simulink model "omav_old_allocation"  (R2020a)
settings: Solver=VariableStepAuto  StartTime=0.0  StopTime=15  RelTol=1e-3
undefined symbols (not defined in the file): params
libraries: simulink x12, vrlib x2
settings Model: Creator=daniel  LastModifiedBy=daniel

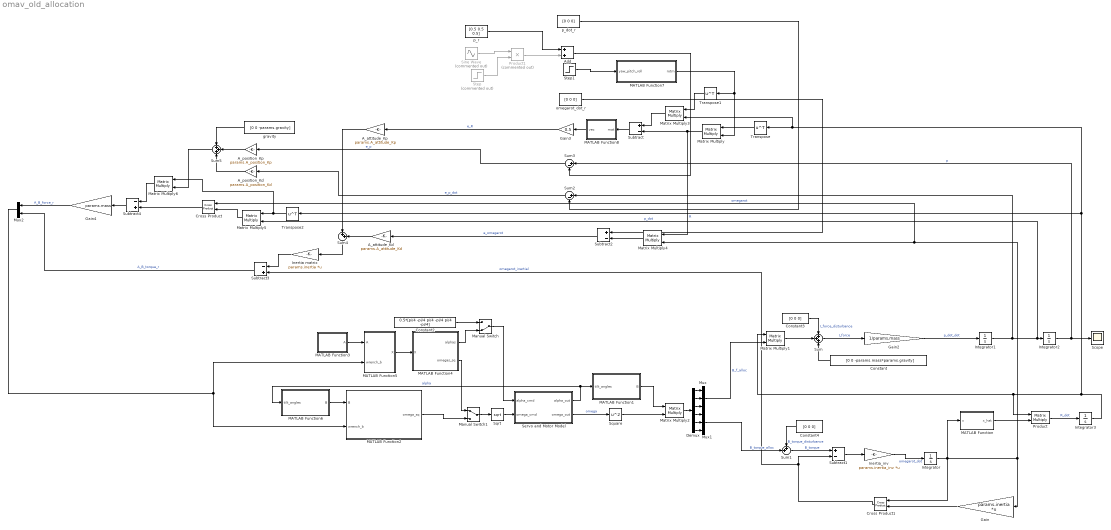
== system omav_old_allocation ==
  A_attitude_Kd : Gain  Gain=params.A_attitude_Kd
  A_attitude_Kp : Gain  Gain=params.A_attitude_Kp
  A_position_Kd : Gain  Gain=params.A_position_Kd
  A_position_Kp : Gain  Gain=params.A_position_Kp
  Add : Sum
  Constant : Constant  Value=[0 0 -params.mass*params.gravity]
  Constant2 : Constant  Value=0.5*[pi/4 -pi/4 pi/4 -pi/4 pi/4 -pi/4]
  Constant3 : Constant  Value=[0 0 0]
  Constant4 : Constant  Value=[0 0 0]
  Cross Product : vrlib/Utilities/Cross Product
  Cross Product1 : vrlib/Utilities/Cross Product
  Demux : Demux  Outputs=6
  Gain : Gain  Gain=params.inertia  Multiplication=Matrix(K*u) (u vector)
  Gain2 : Gain  Gain=1/params.mass
  Gain3 : Gain  Gain=0.5
  Gain4 : Gain  Gain=params.mass
  Inertia matrix : Gain  Gain=params.inertia  Multiplication=Matrix(K*u) (u vector)
  Inertia_inv : Gain  Gain=params.inertia_inv  Multiplication=Matrix(K*u) (u vector)
  Integrator : Integrator
  Integrator1 : Integrator
  Integrator2 : Integrator
  Integrator3 : Integrator  InitialCondition=[1 0 0;0 1 0;0 0 1]
  MATLAB Function : MATLAB Function  TreatAsAtomicUnit=on
  MATLAB Function1 : MATLAB Function  TreatAsAtomicUnit=on
  MATLAB Function2 : MATLAB Function  TreatAsAtomicUnit=on
  MATLAB Function3 : MATLAB Function  TreatAsAtomicUnit=on
  MATLAB Function4 : MATLAB Function  TreatAsAtomicUnit=on
  MATLAB Function5 : MATLAB Function  TreatAsAtomicUnit=on
  MATLAB Function6 : MATLAB Function  TreatAsAtomicUnit=on
  MATLAB Function7 : MATLAB Function  TreatAsAtomicUnit=on
  MATLAB Function8 : MATLAB Function  TreatAsAtomicUnit=on
  Manual Switch : ManualSwitch  CurrentSetting=0
  Manual Switch1 : ManualSwitch
  Matrix Multiply{,1..6} (7 alike) : Product  Multiplication=Matrix(*)
  Mux : Mux  Inputs=3
  Mux1 : Mux  Inputs=3
  Mux2 : Mux  Inputs=2
  Product : Product  Multiplication=Matrix(*)  OutMin=0
  Product1 : Product  Commented=on
  Scope : Scope
  Servo and Motor Model : Subsystem
  Sine Wave : Sin  Commented=on  Amplitude=[0.01 0 0]  Frequency=5  SampleTime=0
  Sqrt : Sqrt  SaturateOnIntegerOverflow=on
  Square : Math  Operator=square  SaturateOnIntegerOverflow=on
  Step : Step  Commented=on  Time=3  SampleTime=0
  Step1 : Step  Time=5  Before=[0 0 0]  After=[0 pi/2 0]  SampleTime=0
  Subtract : Sum  Inputs=+-
  Subtract1 : Sum  Inputs=+-
  Subtract2 : Sum  Inputs=+-
  Subtract3 : Sum  Inputs=-+
  Subtract4 : Sum  Inputs=-+
  Sum : Sum  Inputs=+++
  Sum1 : Sum  Inputs=++|
  Sum2 : Sum  Inputs=|+-
  Sum3 : Sum  Inputs=|+-
  Sum4 : Sum  Inputs=|++
  Sum5 : Sum  Inputs=+++
  Transpose : Math  Operator=transpose  SaturateOnIntegerOverflow=on
  Transpose1 : Math  Operator=transpose  SaturateOnIntegerOverflow=on
  Transpose2 : Math  Operator=transpose  SaturateOnIntegerOverflow=on
  gravity : Constant  Value=[0 0 -params.gravity]
  omegarot_dot_r : Constant  Value=[0 0 0]
  p_dot_r : Constant  Value=[0 0 0]
  p_r : Constant  Value=[0.5 0.5 0.5]
  wires:
  Integrator1/1 -> Matrix Multiply5/2, Integrator2/1, Sum2/1  "p_dot"
  Integrator2/1 -> Sum3/1, Scope/1  "p"
  Gain2/1 -> Integrator1/1  "p_dot_dot"
  Integrator/1 -> Cross Product/1, Matrix Multiply4/2, Gain/1, MATLAB Function/1(x), Cross Product1/1  "omegarot"
  Subtract1/1 -> Inertia_inv/1
  Gain/1 -> Cross Product1/2
  Cross Product1/1 -> Subtract3/2, Subtract1/2  "omegarot_inertial"
  Inertia_inv/1 -> Integrator/1  "omegarot_dot"
  Mux1/1 -> Sum1/2  "B_torque_alloc"
  Sum/1 -> Gain2/1  "I_force"
  MATLAB Function/1(x_hat) -> Product/2
  Integrator3/1 -> Matrix Multiply3/2, Transpose/1, Transpose2/1, Product/1, Matrix Multiply1/1  "R"
  Product/1 -> Integrator3/1  "R_dot"
  Constant3/1 -> Sum/1  "I_force_disturbance"
  Mux/1 -> Matrix Multiply1/2  "B_f_alloc"
  Matrix Multiply1/1 -> Sum/2
  Constant/1 -> Sum/3
  Sum1/1 -> Subtract1/1  "B_torque"
  Constant4/1 -> Sum1/1  "B_torque_disturbance"
  MATLAB Function1/1(B) -> Matrix Multiply2/1
  Matrix Multiply2/1 -> Demux/1
  Demux/1 -> Mux/1
  Demux/2 -> Mux/2
  Demux/3 -> Mux/3
  Demux/5 -> Mux1/2
  Demux/4 -> Mux1/1
  Demux/6 -> Mux1/3
  Servo and Motor Model/1(alpha_out) -> MATLAB Function6/1(tilt_angles), MATLAB Function1/1(tilt_angles)  "alpha"
  Servo and Motor Model/2(omega_out) -> Square/1  "omega"
  Square/1 -> Matrix Multiply2/2
  MATLAB Function2/1(omega_sq) -> Manual Switch1/2
  Sqrt/1 -> Servo and Motor Model/2(omega_cmd)
  MATLAB Function3/1(A) -> MATLAB Function5/1(A)
  MATLAB Function5/1(X) -> MATLAB Function4/1(X)
  MATLAB Function6/1(B) -> MATLAB Function2/1(B)
  MATLAB Function4/1(alphas) -> Manual Switch/2
  Manual Switch/1 -> Servo and Motor Model/1(alpha_cmd)
  Constant2/1 -> Manual Switch/1
  p_dot_r/1 -> Sum2/2
  Sum2/1 -> A_position_Kd/1  "e_p_dot"
  Sum3/1 -> A_position_Kp/1  "e_p"
  Add/1 -> Sum3/2
  Step1/1 -> MATLAB Function7/1(yaw_pitch_roll)
  MATLAB Function7/1(rotm) -> Matrix Multiply/2, Transpose1/1
  Matrix Multiply/1 -> Subtract/2, Matrix Multiply4/1
  Transpose/1 -> Matrix Multiply/1
  Transpose1/1 -> Matrix Multiply3/1
  Matrix Multiply3/1 -> Subtract/1
  Subtract/1 -> MATLAB Function8/1(mat)
  MATLAB Function8/1(vec) -> Gain3/1
  Gain3/1 -> A_attitude_Kp/1  "e_R"
  omegarot_dot_r/1 -> Subtract2/1
  Matrix Multiply4/1 -> Subtract2/2
  Subtract2/1 -> A_attitude_Kd/1  "e_omegarot"
  A_attitude_Kd/1 -> Sum4/2
  A_attitude_Kp/1 -> Sum4/1
  Sum4/1 -> Inertia matrix/1
  Inertia matrix/1 -> Subtract3/1
  Subtract3/1 -> Mux2/2  "A_B_torque_r"
  Transpose2/1 -> Matrix Multiply6/1, Matrix Multiply5/1
  Matrix Multiply5/1 -> Cross Product/2
  A_position_Kp/1 -> Sum5/2
  gravity/1 -> Sum5/1
  A_position_Kd/1 -> Sum5/3
  Sum5/1 -> Matrix Multiply6/2
  Matrix Multiply6/1 -> Subtract4/1
  Cross Product/1 -> Subtract4/2
  Subtract4/1 -> Gain4/1
  Gain4/1 -> Mux2/1  "A_B_force_r"
  Mux2/1 -> MATLAB Function5/2(wrench_b), MATLAB Function2/2(wrench_b)
  Manual Switch1/1 -> Sqrt/1
  MATLAB Function4/2(omegas_sq) -> Manual Switch1/1
  Step/1 -> Product1/2
  Sine Wave/1 -> Product1/1
  Product1/1 -> Add/2
  p_r/1 -> Add/1

== system omav_old_allocation/Servo and Motor Model ==
  alpha_cmd : Inport
  omega_cmd : Inport  Port=2
  all_rotors_subsystem1 : Subsystem
      mask Display: image('images/brushless.JPG'); % Use "Edit Image" on toolstrip to change.
  all_servos_subsystem1 : Subsystem
      mask Display: image('images/servo.jpg'); % Use "Edit Image" on toolstrip to change.
  alpha_out : Outport
  omega_out : Outport  Port=2
  wires:
  alpha_cmd/1 -> all_servos_subsystem1/1(alphas_cmd)  "alpha_cmd"
  all_rotors_subsystem1/1(omegas_out) -> omega_out/1  "omega_out"
  all_servos_subsystem1/1(alphas_out) -> alpha_out/1  "alpha_out"
  omega_cmd/1 -> all_rotors_subsystem1/1(omegas_cmd)  "omega_cmd"

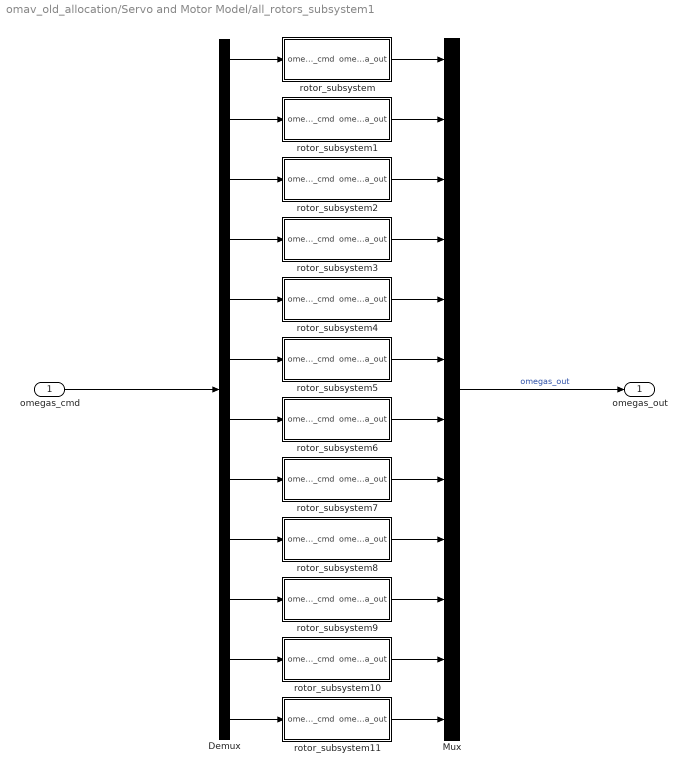
== system omav_old_allocation/Servo and Motor Model/all_rotors_subsystem1 ==
  omegas_cmd : Inport
  Demux : Demux  Outputs=12
  Mux : Mux  Inputs=12
  rotor_subsystem : Subsystem
  rotor_subsystem1 : Subsystem
  rotor_subsystem10 : Subsystem
  rotor_subsystem11 : Subsystem
  rotor_subsystem2 : Subsystem
  rotor_subsystem3 : Subsystem
  rotor_subsystem4 : Subsystem
  rotor_subsystem5 : Subsystem
  rotor_subsystem6 : Subsystem
  rotor_subsystem7 : Subsystem
  rotor_subsystem8 : Subsystem
  rotor_subsystem9 : Subsystem
  omegas_out : Outport
  wires:
  Demux/3 -> rotor_subsystem2/1(omega_cmd)
  rotor_subsystem10/1(omega_out) -> Mux/11
  rotor_subsystem7/1(omega_out) -> Mux/8
  rotor_subsystem2/1(omega_out) -> Mux/3
  rotor_subsystem1/1(omega_out) -> Mux/2
  Demux/2 -> rotor_subsystem1/1(omega_cmd)
  rotor_subsystem5/1(omega_out) -> Mux/6
  rotor_subsystem4/1(omega_out) -> Mux/5
  Demux/4 -> rotor_subsystem3/1(omega_cmd)
  rotor_subsystem6/1(omega_out) -> Mux/7
  Demux/8 -> rotor_subsystem7/1(omega_cmd)
  rotor_subsystem/1(omega_out) -> Mux/1
  rotor_subsystem3/1(omega_out) -> Mux/4
  rotor_subsystem11/1(omega_out) -> Mux/12
  rotor_subsystem8/1(omega_out) -> Mux/9
  Demux/11 -> rotor_subsystem10/1(omega_cmd)
  rotor_subsystem9/1(omega_out) -> Mux/10
  Demux/1 -> rotor_subsystem/1(omega_cmd)
  omegas_cmd/1 -> Demux/1
  Mux/1 -> omegas_out/1  "omegas_out"
  Demux/12 -> rotor_subsystem11/1(omega_cmd)
  Demux/10 -> rotor_subsystem9/1(omega_cmd)
  Demux/9 -> rotor_subsystem8/1(omega_cmd)
  Demux/7 -> rotor_subsystem6/1(omega_cmd)
  Demux/6 -> rotor_subsystem5/1(omega_cmd)
  Demux/5 -> rotor_subsystem4/1(omega_cmd)

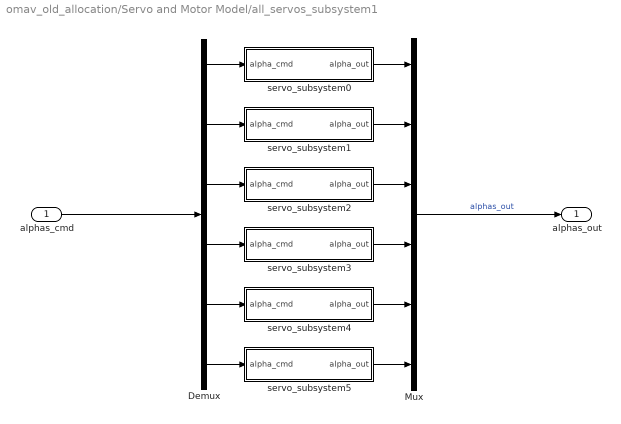
== system omav_old_allocation/Servo and Motor Model/all_servos_subsystem1 ==
  alphas_cmd : Inport
  Demux : Demux  Outputs=6
  Mux : Mux  Inputs=6
  servo_subsystem0 : Subsystem
  servo_subsystem1 : Subsystem
  servo_subsystem2 : Subsystem
  servo_subsystem3 : Subsystem
  servo_subsystem4 : Subsystem
  servo_subsystem5 : Subsystem
  alphas_out : Outport
  wires:
  alphas_cmd/1 -> Demux/1
  Demux/2 -> servo_subsystem1/1(alpha_cmd)
  servo_subsystem3/1(alpha_out) -> Mux/4
  servo_subsystem1/1(alpha_out) -> Mux/2
  Demux/4 -> servo_subsystem3/1(alpha_cmd)
  servo_subsystem4/1(alpha_out) -> Mux/5
  Demux/5 -> servo_subsystem4/1(alpha_cmd)
  Demux/1 -> servo_subsystem0/1(alpha_cmd)
  servo_subsystem2/1(alpha_out) -> Mux/3
  servo_subsystem5/1(alpha_out) -> Mux/6
  Demux/6 -> servo_subsystem5/1(alpha_cmd)
  Demux/3 -> servo_subsystem2/1(alpha_cmd)
  Mux/1 -> alphas_out/1  "alphas_out"
  servo_subsystem0/1(alpha_out) -> Mux/1

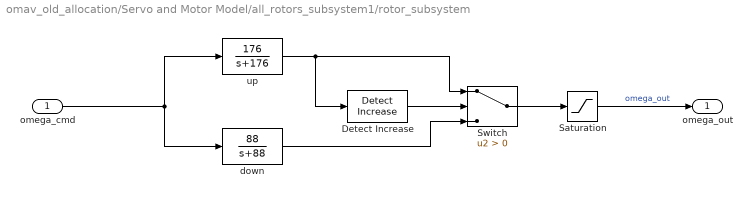
== system omav_old_allocation/Servo and Motor Model/all_rotors_subsystem1/rotor_subsystem ==
  omega_cmd : Inport
  Detect Increase : simulink/Logic and Bit Operations/Detect Increase  vinit=0.0  OutDataTypeStr=boolean
  Saturation : Saturate  UpperLimit=params.rotor_max  LowerLimit=0
  Switch : Switch  Criteria=u2 > Threshold
  down : TransferFcn  Numerator=[88]  Denominator=[1 88]
  up : TransferFcn  Numerator=[176]  Denominator=[1 176]
  omega_out : Outport
  wires:
  down/1 -> Switch/3
  up/1 -> Detect Increase/1, Switch/1
  omega_cmd/1 -> up/1, down/1
  Switch/1 -> Saturation/1
  Detect Increase/1 -> Switch/2
  Saturation/1 -> omega_out/1  "omega_out"

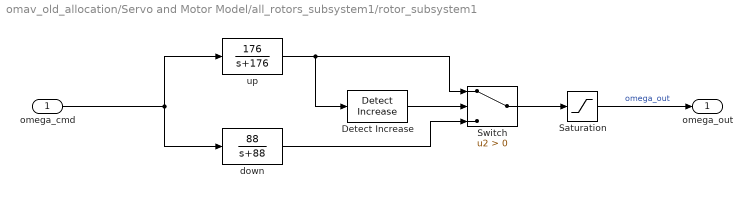
== system omav_old_allocation/Servo and Motor Model/all_rotors_subsystem1/rotor_subsystem1 ==
  omega_cmd : Inport
  Detect Increase : simulink/Logic and Bit Operations/Detect Increase  vinit=0.0  OutDataTypeStr=boolean
  Saturation : Saturate  UpperLimit=params.rotor_max  LowerLimit=0
  Switch : Switch  Criteria=u2 > Threshold
  down : TransferFcn  Numerator=[88]  Denominator=[1 88]
  up : TransferFcn  Numerator=[176]  Denominator=[1 176]
  omega_out : Outport
  wires:
  Saturation/1 -> omega_out/1  "omega_out"
  Detect Increase/1 -> Switch/2
  Switch/1 -> Saturation/1
  omega_cmd/1 -> down/1, up/1
  up/1 -> Switch/1, Detect Increase/1
  down/1 -> Switch/3

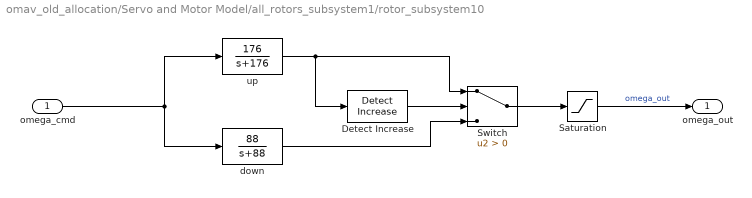
== system omav_old_allocation/Servo and Motor Model/all_rotors_subsystem1/rotor_subsystem10 ==
  omega_cmd : Inport
  Detect Increase : simulink/Logic and Bit Operations/Detect Increase  vinit=0.0  OutDataTypeStr=boolean
  Saturation : Saturate  UpperLimit=params.rotor_max  LowerLimit=0
  Switch : Switch  Criteria=u2 > Threshold
  down : TransferFcn  Numerator=[88]  Denominator=[1 88]
  up : TransferFcn  Numerator=[176]  Denominator=[1 176]
  omega_out : Outport
  wires:
  down/1 -> Switch/3
  up/1 -> Detect Increase/1, Switch/1
  omega_cmd/1 -> up/1, down/1
  Switch/1 -> Saturation/1
  Detect Increase/1 -> Switch/2
  Saturation/1 -> omega_out/1  "omega_out"

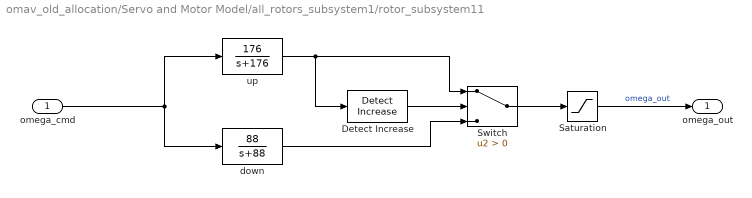
== system omav_old_allocation/Servo and Motor Model/all_rotors_subsystem1/rotor_subsystem11 ==
  omega_cmd : Inport
  Detect Increase : simulink/Logic and Bit Operations/Detect Increase  vinit=0.0  OutDataTypeStr=boolean
  Saturation : Saturate  UpperLimit=params.rotor_max  LowerLimit=0
  Switch : Switch  Criteria=u2 > Threshold
  down : TransferFcn  Numerator=[88]  Denominator=[1 88]
  up : TransferFcn  Numerator=[176]  Denominator=[1 176]
  omega_out : Outport
  wires:
  Saturation/1 -> omega_out/1  "omega_out"
  Detect Increase/1 -> Switch/2
  Switch/1 -> Saturation/1
  omega_cmd/1 -> down/1, up/1
  up/1 -> Switch/1, Detect Increase/1
  down/1 -> Switch/3

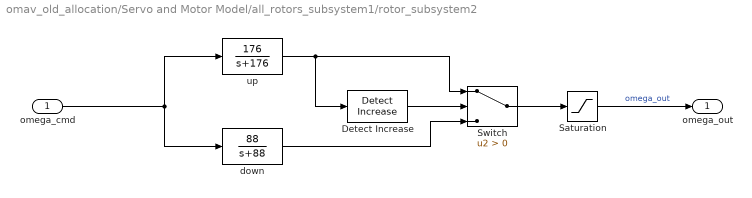
== system omav_old_allocation/Servo and Motor Model/all_rotors_subsystem1/rotor_subsystem2 ==
  omega_cmd : Inport
  Detect Increase : simulink/Logic and Bit Operations/Detect Increase  vinit=0.0  OutDataTypeStr=boolean
  Saturation : Saturate  UpperLimit=params.rotor_max  LowerLimit=0
  Switch : Switch  Criteria=u2 > Threshold
  down : TransferFcn  Numerator=[88]  Denominator=[1 88]
  up : TransferFcn  Numerator=[176]  Denominator=[1 176]
  omega_out : Outport
  wires:
  down/1 -> Switch/3
  up/1 -> Detect Increase/1, Switch/1
  omega_cmd/1 -> up/1, down/1
  Switch/1 -> Saturation/1
  Detect Increase/1 -> Switch/2
  Saturation/1 -> omega_out/1  "omega_out"

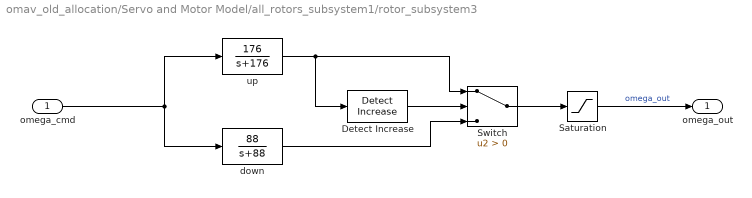
== system omav_old_allocation/Servo and Motor Model/all_rotors_subsystem1/rotor_subsystem3 ==
  omega_cmd : Inport
  Detect Increase : simulink/Logic and Bit Operations/Detect Increase  vinit=0.0  OutDataTypeStr=boolean
  Saturation : Saturate  UpperLimit=params.rotor_max  LowerLimit=0
  Switch : Switch  Criteria=u2 > Threshold
  down : TransferFcn  Numerator=[88]  Denominator=[1 88]
  up : TransferFcn  Numerator=[176]  Denominator=[1 176]
  omega_out : Outport
  wires:
  Saturation/1 -> omega_out/1  "omega_out"
  Detect Increase/1 -> Switch/2
  Switch/1 -> Saturation/1
  omega_cmd/1 -> down/1, up/1
  up/1 -> Switch/1, Detect Increase/1
  down/1 -> Switch/3

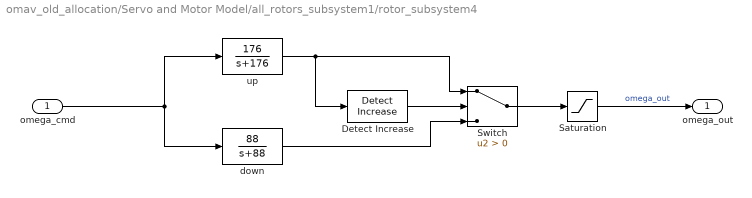
== system omav_old_allocation/Servo and Motor Model/all_rotors_subsystem1/rotor_subsystem4 ==
  omega_cmd : Inport
  Detect Increase : simulink/Logic and Bit Operations/Detect Increase  vinit=0.0  OutDataTypeStr=boolean
  Saturation : Saturate  UpperLimit=params.rotor_max  LowerLimit=0
  Switch : Switch  Criteria=u2 > Threshold
  down : TransferFcn  Numerator=[88]  Denominator=[1 88]
  up : TransferFcn  Numerator=[176]  Denominator=[1 176]
  omega_out : Outport
  wires:
  down/1 -> Switch/3
  up/1 -> Detect Increase/1, Switch/1
  omega_cmd/1 -> up/1, down/1
  Switch/1 -> Saturation/1
  Detect Increase/1 -> Switch/2
  Saturation/1 -> omega_out/1  "omega_out"

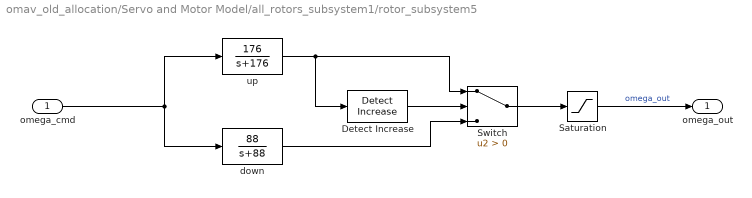
== system omav_old_allocation/Servo and Motor Model/all_rotors_subsystem1/rotor_subsystem5 ==
  omega_cmd : Inport
  Detect Increase : simulink/Logic and Bit Operations/Detect Increase  vinit=0.0  OutDataTypeStr=boolean
  Saturation : Saturate  UpperLimit=params.rotor_max  LowerLimit=0
  Switch : Switch  Criteria=u2 > Threshold
  down : TransferFcn  Numerator=[88]  Denominator=[1 88]
  up : TransferFcn  Numerator=[176]  Denominator=[1 176]
  omega_out : Outport
  wires:
  Saturation/1 -> omega_out/1  "omega_out"
  Detect Increase/1 -> Switch/2
  Switch/1 -> Saturation/1
  omega_cmd/1 -> down/1, up/1
  up/1 -> Switch/1, Detect Increase/1
  down/1 -> Switch/3

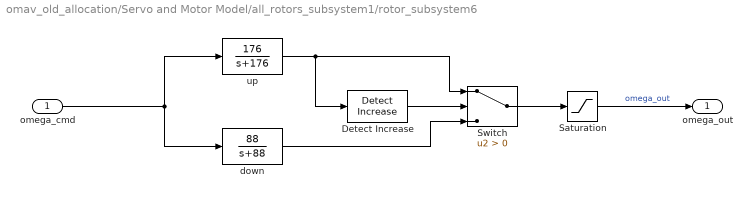
== system omav_old_allocation/Servo and Motor Model/all_rotors_subsystem1/rotor_subsystem6 ==
  omega_cmd : Inport
  Detect Increase : simulink/Logic and Bit Operations/Detect Increase  vinit=0.0  OutDataTypeStr=boolean
  Saturation : Saturate  UpperLimit=params.rotor_max  LowerLimit=0
  Switch : Switch  Criteria=u2 > Threshold
  down : TransferFcn  Numerator=[88]  Denominator=[1 88]
  up : TransferFcn  Numerator=[176]  Denominator=[1 176]
  omega_out : Outport
  wires:
  down/1 -> Switch/3
  up/1 -> Detect Increase/1, Switch/1
  omega_cmd/1 -> up/1, down/1
  Switch/1 -> Saturation/1
  Detect Increase/1 -> Switch/2
  Saturation/1 -> omega_out/1  "omega_out"

== system omav_old_allocation/Servo and Motor Model/all_rotors_subsystem1/rotor_subsystem7 ==
  omega_cmd : Inport
  Detect Increase : simulink/Logic and Bit Operations/Detect Increase  vinit=0.0  OutDataTypeStr=boolean
  Saturation : Saturate  UpperLimit=params.rotor_max  LowerLimit=0
  Switch : Switch  Criteria=u2 > Threshold
  down : TransferFcn  Numerator=[88]  Denominator=[1 88]
  up : TransferFcn  Numerator=[176]  Denominator=[1 176]
  omega_out : Outport
  wires:
  Saturation/1 -> omega_out/1  "omega_out"
  Detect Increase/1 -> Switch/2
  Switch/1 -> Saturation/1
  omega_cmd/1 -> down/1, up/1
  up/1 -> Switch/1, Detect Increase/1
  down/1 -> Switch/3

== system omav_old_allocation/Servo and Motor Model/all_rotors_subsystem1/rotor_subsystem8 ==
  omega_cmd : Inport
  Detect Increase : simulink/Logic and Bit Operations/Detect Increase  vinit=0.0  OutDataTypeStr=boolean
  Saturation : Saturate  UpperLimit=params.rotor_max  LowerLimit=0
  Switch : Switch  Criteria=u2 > Threshold
  down : TransferFcn  Numerator=[88]  Denominator=[1 88]
  up : TransferFcn  Numerator=[176]  Denominator=[1 176]
  omega_out : Outport
  wires:
  down/1 -> Switch/3
  up/1 -> Detect Increase/1, Switch/1
  omega_cmd/1 -> up/1, down/1
  Switch/1 -> Saturation/1
  Detect Increase/1 -> Switch/2
  Saturation/1 -> omega_out/1  "omega_out"

== system omav_old_allocation/Servo and Motor Model/all_rotors_subsystem1/rotor_subsystem9 ==
  omega_cmd : Inport
  Detect Increase : simulink/Logic and Bit Operations/Detect Increase  vinit=0.0  OutDataTypeStr=boolean
  Saturation : Saturate  UpperLimit=params.rotor_max  LowerLimit=0
  Switch : Switch  Criteria=u2 > Threshold
  down : TransferFcn  Numerator=[88]  Denominator=[1 88]
  up : TransferFcn  Numerator=[176]  Denominator=[1 176]
  omega_out : Outport
  wires:
  Saturation/1 -> omega_out/1  "omega_out"
  Detect Increase/1 -> Switch/2
  Switch/1 -> Saturation/1
  omega_cmd/1 -> down/1, up/1
  up/1 -> Switch/1, Detect Increase/1
  down/1 -> Switch/3

== system omav_old_allocation/Servo and Motor Model/all_servos_subsystem1/servo_subsystem0 ==
  alpha_cmd : Inport
  Servo Transfer Function : TransferFcn  Numerator=[256]  Denominator=[1 22.4 256]
  alpha_out : Outport
  wires:
  alpha_cmd/1 -> Servo Transfer Function/1
  Servo Transfer Function/1 -> alpha_out/1  "alpha_out"

== system omav_old_allocation/Servo and Motor Model/all_servos_subsystem1/servo_subsystem1 ==
  alpha_cmd : Inport
  Servo Transfer Function : TransferFcn  Numerator=[256]  Denominator=[1 22.4 256]
  alpha_out : Outport
  wires:
  Servo Transfer Function/1 -> alpha_out/1  "alpha_out"
  alpha_cmd/1 -> Servo Transfer Function/1

== system omav_old_allocation/Servo and Motor Model/all_servos_subsystem1/servo_subsystem2 ==
  alpha_cmd : Inport
  Servo Transfer Function : TransferFcn  Numerator=[256]  Denominator=[1 22.4 256]
  alpha_out : Outport
  wires:
  alpha_cmd/1 -> Servo Transfer Function/1
  Servo Transfer Function/1 -> alpha_out/1  "alpha_out"

== system omav_old_allocation/Servo and Motor Model/all_servos_subsystem1/servo_subsystem3 ==
  alpha_cmd : Inport
  Servo Transfer Function : TransferFcn  Numerator=[256]  Denominator=[1 22.4 256]
  alpha_out : Outport
  wires:
  Servo Transfer Function/1 -> alpha_out/1  "alpha_out"
  alpha_cmd/1 -> Servo Transfer Function/1

== system omav_old_allocation/Servo and Motor Model/all_servos_subsystem1/servo_subsystem4 ==
  alpha_cmd : Inport
  Servo Transfer Function : TransferFcn  Numerator=[256]  Denominator=[1 22.4 256]
  alpha_out : Outport
  wires:
  alpha_cmd/1 -> Servo Transfer Function/1
  Servo Transfer Function/1 -> alpha_out/1  "alpha_out"

== system omav_old_allocation/Servo and Motor Model/all_servos_subsystem1/servo_subsystem5 ==
  alpha_cmd : Inport
  Servo Transfer Function : TransferFcn  Numerator=[256]  Denominator=[1 22.4 256]
  alpha_out : Outport
  wires:
  Servo Transfer Function/1 -> alpha_out/1  "alpha_out"
  alpha_cmd/1 -> Servo Transfer Function/1

== matlab function omav_old_allocation/MATLAB Function ==
  data: x input; x_hat output
function x_hat = hat_map(x)
x_hat = [0 -x(3) x(2); x(3) 0 -x(1); -x(2) x(1) 0];

== matlab function omav_old_allocation/MATLAB Function2 ==
  data: B input; omega_sq output; wrench_b input
function omega_sq = get_omegasq(B,wrench_b)
%GET_OMEGASQ Summary of this function goes here
%   Detailed explanation goes here

params = parameters();
omega_sq = pinv(B)*wrench_b;

for i = 1:12
    if omega_sq(i) < 0
        omega_sq(i) = 0;
    end
    
    if omega_sq(i) > (params.rotor_max)^2
        omega_sq(i) = (params.rotor_max)^2;
    end
end

end

== matlab function omav_old_allocation/MATLAB Function3 ==
  data: A output
function A = get_A()
%[F, tau] = A * [sin(alpha)*omega², cos(alpha)*omega²]

params = parameters();

rotor_force_constant = params.rotor_force_constant;
rotor_moment_constant = params.rotor_moment_constant;
arm_length = params.arm_length;

arm_angles = params.arm_angles;
spin = params.spin;

%implementing pre-calculated matrix
%zero entries are commented out
A = zeros(6,24);

%iterating through every rotor
%refactored to z-up coordinate system
for i = 1:12
    A(1,2*i-1) = sin(arm_angles(i));
    %A(1,2*i) = 0;
    
    A(2,2*i-1) = -cos(arm_angles(i));
    %A(2,2*i) = 0;
    
    %A(3,2*i-1) = 0;
    A(3,2*i) = 1;
    
    A(4,2*i-1) = -rotor_moment_constant*spin(i)*sin(arm_angles(i));
    A(4,2*i) = sin(arm_angles(i))*arm_length;
    
    A(5,2*i-1) = rotor_moment_constant*spin(i)*cos(arm_angles(i));
    A(5,2*i) = -cos(arm_angles(i))*arm_length;
    
    A(6,2*i-1) = -arm_length;
    A(6,2*i) = -rotor_moment_constant*spin(i);
end

%multiplying with rotor force constant
A = A*rotor_force_constant;

== matlab function omav_old_allocation/MATLAB Function4 ==
  data: X input; alphas output; omegas_sq output
function [alphas, omegas_sq] = get_projections(X)
%GET_PROJECTIONS Summary of this function goes here
%   Detailed explanation goes here


%get the angles
alphas = zeros(6,1);
for i = 1:6
    %get to entry which corresponds to arm
    j = 4*i - 3;
    alphas(i) = atan2(X(j)+X(j+2),X(j+1)+X(j+3));
end

omegas_sq = zeros(12,1);
for i = 1:6
    %get to entry which corresponds to arm
    j = 4*i - 3;
    
    omegas_sq(2*i-1) = X(j)*sin(alphas(i)) + X(j+1)*cos(alphas(i));
    omegas_sq(2*i)   = X(j+2)*sin(alphas(i)) + X(j+3)*cos(alphas(i));
end

%set to zero if smaller than zero
for i = 1:12
    if omegas_sq(i) < 0
        omegas_sq(i) = 0;
    end
end

== matlab function omav_old_allocation/MATLAB Function5 ==
  data: A input; X output; wrench_b input
function X = get_X(A,wrench_b)
%GET_X Summary of this function goes here
%   Detailed explanation goes here
wrench_b = wrench_b(:);

X = pinv(A)*wrench_b;
end

== matlab function omav_old_allocation/MATLAB Function6 ==
  data: tilt_angles input; B output
function B = get_B(tilt_angles)
%tilt_angles [6x1]
%[F, tau] = B * [omega²]

params = parameters();

rotor_force_constant = params.rotor_force_constant;
rotor_moment_constant = params.rotor_moment_constant;
arm_length = params.arm_length;

arm_angles = params.arm_angles;
spin = params.spin;

B = zeros(6,12);


j = 0;

%repeat every tilt angle
rep_tilt_angles = repelem(tilt_angles,2);
%iterating through every rotor
%refactored to z-upwards
for i = 1:12
  
    tilt_angle = rep_tilt_angles(i);
    
    B(1,i) = sin(arm_angles(i))*sin(tilt_angle);
    B(2,i) = -cos(arm_angles(i))*sin(tilt_angle);
    B(3,i) = cos(tilt_angle);
    B(4,i) = -(rotor_moment_constant*spin(i)*sin(tilt_angle) - cos(tilt_angle)*arm_length)*sin(arm_angles(i));
    B(5,i) =  (rotor_moment_constant*spin(i)*sin(tilt_angle) - cos(tilt_angle)*arm_length)*cos(arm_angles(i));
    B(6,i) = -(rotor_moment_constant*spin(i)*cos(tilt_angle) + sin(tilt_angle)*arm_length);
end

B = B*rotor_force_constant;

== matlab function omav_old_allocation/MATLAB Function7 ==
  data: yaw_pitch_roll input; rotm output
function rotm = fcn(yaw_pitch_roll)
yaw_pitch_roll = yaw_pitch_roll(:)';
rotm = eul2rotm(yaw_pitch_roll);

== matlab function omav_old_allocation/MATLAB Function8 ==
  data: mat input; vec output
function vec = vee_map(mat)

vec = [-mat(2,3); mat(1,3); -mat(1,2)];

== matlab function omav_old_allocation/MATLAB Function1 ==
  data: tilt_angles input; B output
function B = get_B(tilt_angles)
%tilt_angles [6x1]
%[F, tau] = B * [omega²]

params = parameters();

rotor_force_constant = params.rotor_force_constant;
rotor_moment_constant = params.rotor_moment_constant;
arm_length = params.arm_length;

arm_angles = params.arm_angles;
spin = params.spin;

B = zeros(6,12);


j = 0;

%repeat every tilt angle
rep_tilt_angles = repelem(tilt_angles,2);
%iterating through every rotor
%refactored to z-upwards
for i = 1:12
  
    tilt_angle = rep_tilt_angles(i);
    
    B(1,i) = sin(arm_angles(i))*sin(tilt_angle);
    B(2,i) = -cos(arm_angles(i))*sin(tilt_angle);
    B(3,i) = cos(tilt_angle);
    B(4,i) = -(rotor_moment_constant*spin(i)*sin(tilt_angle) - cos(tilt_angle)*arm_length)*sin(arm_angles(i));
    B(5,i) =  (rotor_moment_constant*spin(i)*sin(tilt_angle) - cos(tilt_angle)*arm_length)*cos(arm_angles(i));
    B(6,i) = -(rotor_moment_constant*spin(i)*cos(tilt_angle) + sin(tilt_angle)*arm_length);
end

B = B*rotor_force_constant;
